simulink model "untitled"  (R2026a)
settings: Solver=FixedStepAuto  StopTime=inf
StopFcn:
  | if exist('out', 'var') && isprop(out, 'driven_pos')
  |     % Case 1: Saved inside 'out' object
  |     writematrix(out.driven_pos.Data, 'driven_waypoints.txt', 'Delimiter', ',');
  | elseif exist('driven_pos', 'var')
  |     % Case 2: Saved directly to Base Workspace
  |     if isa(driven_pos, 'timeseries')
  |         writematrix(driven_pos.Data, 'driven_waypoints.txt', 'Delimiter', ',');
  |     else
  |         writematrix(driven_pos, 'driven_waypoints.txt', 'Delimiter', ',');
  |     end
  | elseif exist('out', 'var') && isprop(out, 'logsout') && ~isempty(out.logsout.get('driven_pos'))
  |     % Case 3: Logged via Signal Logging (logsout)
  |     sigData = out.logsout.get('driven_pos').Values.Data;
  |     writematrix(sigData, 'driven_waypoints.txt', 'Delimiter', ',');
  | else
  |     warning('driven_pos signal not found. Verify To Workspace block settings.');
  | end
undefined symbols (not defined in the file or in its folder): Speed, SteeringAngle
libraries: robotlib x3
settings Model: Creator=prana  LastModifiedBy=prana
settings HardwareCC: ProdHWDeviceType=Generic->Unspecified (assume 32-bit Generic)
settings RTWCC: SystemTargetFile=ert.tlc  HardwareBoard=Robot Operating System (ROS)  TLCOptions="-aInlineSetEventsForThisBaseRateFcn=TLC_FALSE -aSuppressMultiTaskScheduler=TLC_FALSE  -aRateBasedStepFcn=0"  Toolchain=Catkin  TargetLang=C++  Description=Embedded Coder

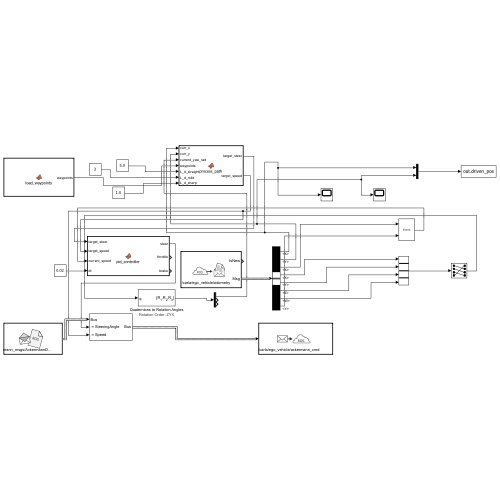
[thumbnail: Simulink's stored preview of the top-level diagram]
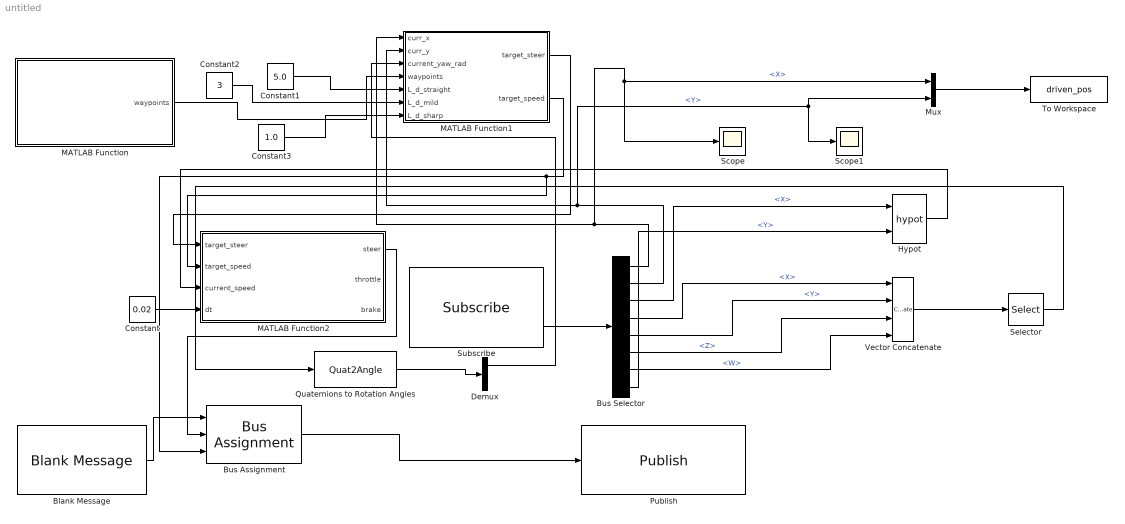
== system untitled ==
  Blank Message : robotlib/Blank Message  messageClass=Message  entityType=ackermann_msgs/AckermannDrive  messageType=ackermann_msgs/AckermannDrive  SampleTime=-1  legacyBusStruct=off
  Bus Assignment : BusAssignment  AssignedSignals=SteeringAngle,Speed
  Bus Selector : BusSelector  OutputSignals=Pose.Pose.Position.X,Pose.Pose.Position.Y,Twist.Twist.Linear.X,Pose.Pose.Orientation.X,Pose.Pose.Orientation.Y,Pose.Pose.Orientation.Z,Pose.Pose.Orientation.W,Twist.Twist.Linear.Y
  Constant : Constant  Value=0.02
  Constant1 : Constant  Value=5.0
  Constant2 : Constant  Value=3
  Constant3 : Constant  Value=1.0
  Demux : Demux  Outputs=3
  Hypot : Math  Operator=hypot
  MATLAB Function : MATLAB Function  TreatAsAtomicUnit=on
  MATLAB Function1 : MATLAB Function  TreatAsAtomicUnit=on
  MATLAB Function2 : MATLAB Function  TreatAsAtomicUnit=on
  Mux : Mux  Inputs=2
  Publish : robotlib/Publish  topicSource=Specify your own  topic=/carla/ego_vehicle/ackermann_cmd  messageType=ackermann_msgs/AckermannDrive  legacyBusStruct=off  messageQueueLength=1
  Quaternions to Rotation Angles : Quat2Angle
      settings: AttributesFormatString=Rotation Order: %<rotationOrder>
  Scope : Scope
      settings: ActiveDisplayYMinimum=-42.169843316078186  ActiveDisplayYMaximum=-2.4768728017807016
  Scope1 : Scope
      settings: ActiveDisplayYMinimum=68.443570137023926  ActiveDisplayYMaximum=102.59444713592529
  Selector : Selector  InputPortWidth=4  IndexOptions=Index vector (dialog)  Indices=[4 1 2 3]  OutputSizes=1
  Subscribe : robotlib/Subscribe  topicSource=Specify your own  topic=/carla/ego_vehicle/odometry  messageType=nav_msgs/Odometry  SampleTime=-1  legacyBusStruct=off  messageQueueLength=1
  To Workspace : ToWorkspace  VariableName=driven_pos  SaveFormat=Timeseries  SampleTime=-1
  Vector Concatenate : Concatenate  NumInputs=4
  wires:
  Subscribe/2 -> Bus Selector/1
  Bus Selector/1 -> Scope/1, Mux/1, MATLAB Function1/1(curr_x)  "<X>"
  Bus Selector/2 -> Scope1/1, Mux/2, MATLAB Function1/2(curr_y)  "<Y>"
  Constant/1 -> MATLAB Function2/4(dt)
  Constant1/1 -> MATLAB Function1/5(L_d_straight)
  MATLAB Function1/1(target_steer) -> MATLAB Function2/1(target_steer)
  MATLAB Function1/2(target_speed) -> Bus Assignment/3, MATLAB Function2/2(target_speed)
  Bus Selector/3 -> Hypot/1  "<X>"
  Bus Selector/8 -> Hypot/2  "<Y>"
  Hypot/1 -> MATLAB Function2/3(current_speed)
  Bus Selector/4 -> Vector Concatenate/1  "<X>"
  Bus Selector/5 -> Vector Concatenate/2  "<Y>"
  Bus Selector/6 -> Vector Concatenate/3  "<Z>"
  Bus Selector/7 -> Vector Concatenate/4  "<W>"
  Quaternions to Rotation Angles/1 -> Demux/1
  Blank Message/1 -> Bus Assignment/1
  Bus Assignment/1 -> Publish/1
  MATLAB Function/1(waypoints) -> MATLAB Function1/4(waypoints)
  Vector Concatenate/1 -> Selector/1
  Selector/1 -> Quaternions to Rotation Angles/1
  Mux/1 -> To Workspace/1
  Demux/1 -> MATLAB Function1/3(current_yaw_rad)
  Constant2/1 -> MATLAB Function1/6(L_d_mild)
  Constant3/1 -> MATLAB Function1/7(L_d_sharp)
  MATLAB Function2/1(steer) -> Bus Assignment/2

== matlab function untitled/MATLAB Function1 ==
  data: curr_x input; target_steer output; curr_y input; current_yaw_rad input; waypoints input double size=[1307 4]; L_d_straight input; target_speed output; L_d_mild input; L_d_sharp input
function [target_steer, target_speed] = process_path(curr_x, curr_y, current_yaw_rad, waypoints, L_d_straight, L_d_mild, L_d_sharp)
    assert(isa(waypoints, 'double'));
    assert(size(waypoints, 1) == 1307);
    assert(size(waypoints, 2) == 4);
    
    persistent last_idx;
    num_pts = size(waypoints, 1);
    
    curr_x = double(curr_x);
    curr_y = double(curr_y);
    current_yaw_rad = double(current_yaw_rad);
    L_d_straight = double(L_d_straight);
    L_d_mild = double(L_d_mild);
    L_d_sharp = double(L_d_sharp);
    
    % 1. Initial Search: Find closest waypoint on first frame
    if isempty(last_idx)
        dx_all = waypoints(:, 1) - curr_x;
        dy_all = waypoints(:, 2) - curr_y;
        dists = sqrt(dx_all.^2 + dy_all.^2);
        [~, min_idx] = min(dists);
        last_idx = min_idx;
    end
    
    % 2. Advance Waypoint Index
    advance_radius = 1.5; % Meters
    while last_idx < num_pts
        dx = waypoints(last_idx, 1) - curr_x;
        dy = waypoints(last_idx, 2) - curr_y;
        if sqrt(dx^2 + dy^2) < advance_radius
            last_idx = last_idx + 1;
        else
            break;
        end
    end
    
    % 3. Curvature Assessment & Decision (Speed & L_d)
    idx_ahead = min(last_idx + 5, num_pts);
    yaw_diff = waypoints(idx_ahead, 4) - waypoints(last_idx, 4);
    curvature = abs(atan2(sin(yaw_diff), cos(yaw_diff)));
    
    % Curvature thresholds (in radians)
    thresh_mild = 0.10;  % ~5.7 degrees heading change
    thresh_sharp = 0.30; % ~17.2 degrees heading change
    
    if curvature < thresh_mild
        % Straight path
        target_speed = single(5.0);
        L_d = L_d_straight;
    elseif curvature < thresh_sharp
        % Mild turn
        target_speed = single(3.0);
        L_d = L_d_mild;
    else
        % Sharp turn
        target_speed = single(1.0);
        L_d = L_d_sharp;
    end
    
    % 4. Select Lookahead Target based on selected L_d
    target_idx = last_idx;
    for i = last_idx:num_pts
        dx = waypoints(i, 1) - curr_x;
        dy = waypoints(i, 2) - curr_y;
        if sqrt(dx^2 + dy^2) >= L_d
            target_idx = i;
            break;
        end
    end
    
    % 5. Pure Pursuit Steering Calculation
    target_x = waypoints(target_idx, 1);
    target_y = waypoints(target_idx, 2);
    
    alpha = atan2(target_y - curr_y, target_x - curr_x) - current_yaw_rad;
    alpha = atan2(sin(alpha), cos(alpha)); % Wrap to [-pi, pi]
    L = 2.875; % Wheelbase from carla_ros_bridge_custom.py
    steer_angle_rad = atan2(2 * L * sin(alpha), L_d);
    
    % CARLA INVERSION: Negate steer_angle_rad so ROS +angle turns CARLA left
    max_steer_rad = 0.70;
    clamped_steer = max(-max_steer_rad, min(max_steer_rad, -steer_angle_rad));
    
    target_steer = single(clamped_steer);
end

== matlab function untitled/MATLAB Function ==
  data: waypoints output double size=[1307 4]
function waypoints = load_waypoints()
    persistent wp_data;
    coder.extrinsic('readmatrix');
    
    if isempty(wp_data)
        % Pre-allocate persistent variable with explicit dimensions (1307x4) and double type
        wp_data = zeros(1307, 4);
        
        % Assign extrinsic readmatrix output directly into the pre-allocated array
        wp_data = readmatrix('waypoints.txt', 'CommentStyle', '#');
    end
    
    waypoints = wp_data;
end

== matlab function untitled/MATLAB Function2 ==
  data: target_steer input; steer output; target_speed input; current_speed input; dt input; throttle output; brake output
function [steer, throttle, brake] = pid_controller(target_steer, target_speed, current_speed, dt)
    % Convert inputs to double for internal operations
    target_speed  = double(target_speed);
    current_speed = double(current_speed);
    dt            = double(dt);

    % --- Longitudinal PID Gains ---
    Kp_v = 0.60; 
    Ki_v = 0.05; 
    Kd_v = 0.02;
    
    persistent int_speed prev_speed_err;
    if isempty(int_speed)
        int_speed = 0.0;
        prev_speed_err = 0.0;
    end
    
    % Steering command directly mapped from Pure Pursuit calculation
    steer = single(target_steer);
    
    % Speed Error Calculation
    error_speed = target_speed - current_speed;
    
    % Speed PID Execution
    int_speed = max(-2.0, min(2.0, int_speed + error_speed * dt)); % Anti-windup
    der_speed = (error_speed - prev_speed_err) / dt;
    prev_speed_err = error_speed;
    u_speed = Kp_v * error_speed + Ki_v * int_speed + Kd_v * der_speed;
    
    % Map Control Output to CARLA Actuator Ranges [0.0, 1.0]
    if u_speed >= 0
        throttle_d = min(1.0, u_speed);
        brake_d = 0.0;
    else
        throttle_d = 0.0;
        brake_d = min(1.0, abs(u_speed));
    end

    throttle = single(throttle_d);
    brake    = single(brake_d);
end
